simulink model "Inciso_b"  (R2024b)
settings: Solver=ode45  StartTime=0.0  StopTime=10.0  RelTol=1e-3
settings Model: Creator=Lenovo  LastModifiedBy=Lenovo

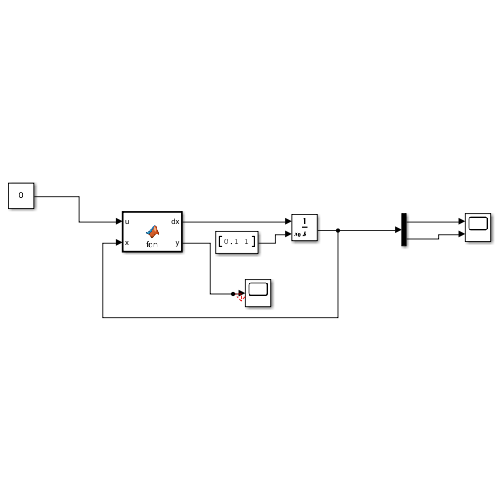
[thumbnail: Simulink's stored preview of the top-level diagram]
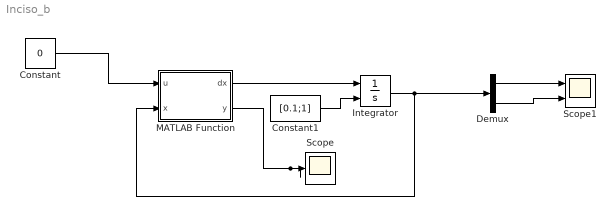
== system Inciso_b ==
  Constant : Constant  Value=0
  Constant1 : Constant  Value=[0.1;1]
  Demux : Demux  Outputs=2
  Integrator : Integrator  InitialConditionSource=external
  MATLAB Function : MATLAB Function  TreatAsAtomicUnit=on
  Scope : Scope
  Scope1 : Scope  NumInputPorts=2
  wires:
  Constant/1 -> MATLAB Function/1(u)
  Integrator/1 -> Demux/1, MATLAB Function/2(x)
  MATLAB Function/1(dx) -> Integrator/1
  Constant1/1 -> Integrator/2
  Demux/1 -> Scope1/1
  Demux/2 -> Scope1/2
  MATLAB Function/2(y) -> Scope/1

== matlab function Inciso_b/MATLAB Function ==
  data: dx output; u input; y output; x input
function [dx, y] = fcn(u,x)

k=2;
b=0.2;
m=1;
x1=x(1);
x2=x(2);
dx1=x2;
dx2=b*x2/m-k*x1/m+u/m;
dx = [dx1;dx2];

y = x1;
